simulink model "AbabilFlightController_Android"  (R2021a)
settings: Solver=ode3  StartTime=0.0  StopTime=40.0  RelTol=1e-3
InitFcn:
  | Ts=0.01
  | kFactor = 1.2;
  | 
  | KpRollAttitude = 0.630138625117681 / kFactor;
  | KiRollAttitude = 0.0552303199591522 / kFactor;
  | 
  | KpPitchAttitude = 0.630138625117681 / kFactor;
  | KiPitchAttitude = 0.0552303199591522 / kFactor;
  | 
  | KpRollRate = 1.31533836563383 / kFactor;
  | KiRollRate = 0.460338699849681 / kFactor;
  | 
  | KpPitchRate = 1.31533836563383 / kFactor;
  | KiPitchRate = 0.460338699849681 / kFactor;
  | 
  | KpYawRate = 1.31533836563383 / kFactor;
  | KiYawRate = 0.460338699849681 / kFactor;
undefined symbols (not defined in the file): Accel, AHRS_Ang_Vel, AHRS_Attitude, Alt, androidSerialSendReceive, AttiudeFiltered, Data_Input, fdesignblkfcn, gcbh, Gyro, kalman, Mag, Static_Orientation
libraries: androiduilib x10, androidsensorlib x5, pid_lib x5, androidcommunicationlib x2, mspfiltlib x1, simulink_extras x1, simulink x1, aerolibatmos2 x1
(part 2 of 2)

== matlab function AbabilFlightController_Android/Flight_Controller/Attitude_Control/pwm_out1 ==
  data: Roll input; M1 output; Pitch input; Yaw input; Thrust input; M2 output; M3 output; M4 output; M5 output; M6 output
function [M1, M2, M3, M4, M5, M6] = motor_mixer(Roll, Pitch, Yaw, Thrust)

idle_PWM = uint16(100);

% Quad X
M1 = uint16(single(((Roll + Pitch - Yaw) / 2 * Thrust + Thrust) * single(100))) + idle_PWM;
M2 = uint16(single(((-Roll + Pitch + Yaw) / 2 * Thrust + Thrust) * single(100))) + idle_PWM;
M3 = uint16(single(((-Roll - Pitch - Yaw) / 2 * Thrust + Thrust) * single(100))) + idle_PWM;
M4 = uint16(single(((Roll - Pitch + Yaw) / 2 * Thrust + Thrust) * single(100))) + idle_PWM;
M5 = 100;
M6 = 100;
M7 = 100;
M8 = 100;

% Quad +
% M1 = ((Pitch - Yaw) * Thrust / 2 + Thrust) * 1000 + idle_PWM;
% M2 = ((-Roll + Yaw) * Thrust / 2 + Thrust) * 1000 + idle_PWM;
% M3 = ((-Pitch - Yaw) * Thrust / 2 + Thrust) * 1000 + idle_PWM;
% M4 = ((Roll + Yaw) * Thrust / 2 + Thrust) * 1000 + idle_PWM;
% M5 = 1000;
% M6 = 1000;
% M7 = 1000;
% M8 = 1000;

% Hex X
% M1 = ((Pitch + Roll / 2 - Yaw) * Thrust / 2 + Thrust) * 1000 + idle_PWM;
% M2 = ((Pitch - Roll / 2 + Yaw) * Thrust / 2 + Thrust) * 1000 + idle_PWM;
% M3 = ((-Roll - Yaw) * Thrust / 2 + Thrust) * 1000 + idle_PWM;
% M4 = ((-Pitch - Roll / 2 + Yaw) * Thrust / 2 + Thrust) * 1000 + idle_PWM;
% M5 = ((-Pitch + Roll / 2 - Yaw) * Thrust / 2 + Thrust) * 1000 + idle_PWM;
% M6 = ((Roll + Yaw) * Thrust / 2 + Thrust) * 1000 + idle_PWM;
% M7 = 1000;
% M8 = 1000;

% Hex X (From Adam)
% M1 = uint16(single(((-Roll - Yaw) * Thrust / 3 + Thrust) * single(1000))) + idle_PWM;
% M2 = uint16(single(((Roll + Yaw) * Thrust / 3 + Thrust) * single(1000))) + idle_PWM;
% M3 = uint16(single(((Pitch + (Roll / 2) - Yaw) * Thrust / 3 + Thrust) * single(1000))) + idle_PWM;
% M4 = uint16(single(((-Pitch - (Roll / 2) + Yaw) * Thrust / 3 + Thrust) * single(1000))) + idle_PWM;
% M5 = uint16(single(((Pitch - (Roll / 2) + Yaw) * Thrust / 3 + Thrust) * single(1000))) + idle_PWM;
% M6 = uint16(single(((-Pitch + (Roll / 2) - Yaw) * Thrust / 3 + Thrust) * single(1000))) + idle_PWM;

% Hex X (Version 2)
% Roll/Yaw
% M1 = ((-Roll - Yaw) * Thrust / 2 + Thrust) * 1000 + idle_PWM;
% M2 = ((Roll + Yaw) * Thrust / 2 + Thrust) * 1000 + idle_PWM;
% % + Pitch/Roll
% M6 = ((Pitch + Roll / 2 - Yaw) * Thrust / 2 + Thrust) * 1000 + idle_PWM;
% M4 = ((Pitch - Roll / 2 + Yaw) * Thrust / 2 + Thrust) * 1000 + idle_PWM;
% % - Pitch/Roll
% M5 = ((-Pitch - Roll / 2 + Yaw) * Thrust / 2 + Thrust) * 1000 + idle_PWM;
% M3 = ((-Pitch + Roll / 2 - Yaw) * Thrust / 2 + Thrust) * 1000 + idle_PWM;

== matlab function AbabilFlightController_Android/Flight_Controller/ExtendedKalamanFilter/EKF ==
  data: Accelerometer input; phi output; Gyroscope input; Magnetometer input; theta output; psi output; dt input
function [phi, theta, psi] = fcn(Accelerometer,Gyroscope,Magnetometer,dt)
persistent AHRSEKF;
if isempty(AHRSEKF)
    AHRSEKF = EKFfilter();
end
    AHRSEKF.Update(dt, Gyroscope(1,:) , Accelerometer(1,:), Magnetometer(1,:));
     phi = AHRSEKF.eulerAngles(1,1);   
     theta = AHRSEKF.eulerAngles(2,1);   
     psi = AHRSEKF.eulerAngles(3,1); 

end

== matlab function AbabilFlightController_Android/Flight_Controller/ExtendedKalamanFilter/MATLAB Function ==
  data: u input; y output
function y = angleCorrection(u)
if u<0
    y = u+6.2832;

else
y = u;
end 
end
